simulink model "Evita_paredes"  (R2023b)
settings: Solver=VariableStepAuto  StartTime=0.0  StopTime=10.0  RelTol=1e-3
settings Model: Creator=Manuel  LastModifiedBy=Manuel

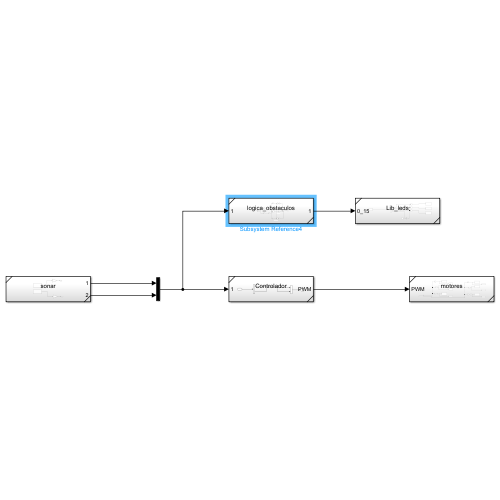
[thumbnail: Simulink's stored preview of the top-level diagram]
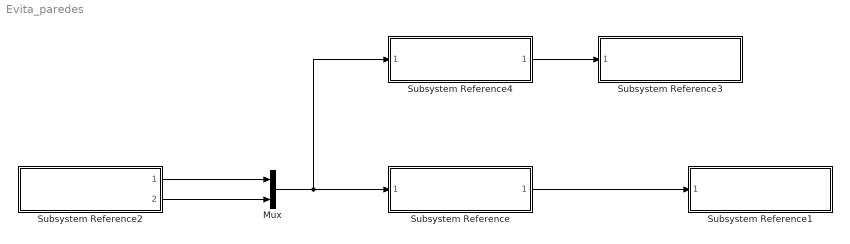
== system Evita_paredes ==
  Mux : Mux  Inputs=2
  Subsystem Reference : Subsystem  ReferencedSubsystem=Controlador
  Subsystem Reference1 : Subsystem  ReferencedSubsystem=motores
  Subsystem Reference2 : Subsystem  ReferencedSubsystem=sonar
  Subsystem Reference3 : Subsystem  ReferencedSubsystem=Lib_leds
  Subsystem Reference4 : Subsystem  ReferencedSubsystem=logica_obstaculos
  wires:
  Subsystem Reference/1 -> Subsystem Reference1/1
  Mux/1 -> Subsystem Reference4/1, Subsystem Reference/1
  Subsystem Reference2/1 -> Mux/1
  Subsystem Reference2/2 -> Mux/2
  Subsystem Reference4/1 -> Subsystem Reference3/1
